simulink model "pwm_sinwave"  (R2015a)
settings: Solver=ode45  StartTime=0.0  StopTime=1  MaxStep=1e-6  RelTol=1e-3
libraries: powerlib x9, simulink x1
settings Model: Creator=KP SINGH  LastModifiedBy=KP SINGH

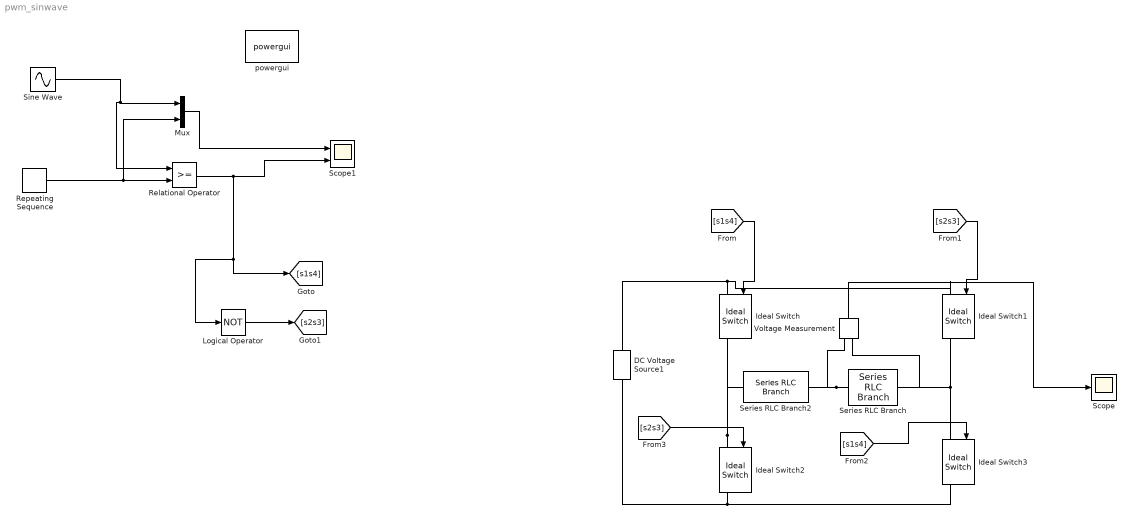
== system pwm_sinwave ==
  DC Voltage Source1 : powerlib/Electrical Sources/DC Voltage Source  Amplitude=100  Measurements=None
  Ideal Switch{,1..3} (4 alike) : powerlib/Power Electronics/Ideal Switch  Ron=0.001  Lon=0  IC=0  Rs=1e5  Cs=inf  Measurements=on
  Logical Operator : Logic  Operator=NOT  IconShape=distinctive  AllPortsSameDT=off  OutDataTypeStr=boolean
  Mux : Mux  Inputs=2
  Relational Operator : RelationalOperator  OutDataTypeStr=boolean
  Repeating Sequence : simulink/Sources/Repeating Sequence  rep_seq_t=[0 1 2 3 4]/10000  rep_seq_y=[0 1 0 -1 0]
  Scope : Scope
      settings: YMin=-100  YMax=100
  Scope1 : Scope  NumInputPorts=2
      settings: YMin=-5~-5  YMax=5~5  MaxDataPoints=5
  Series RLC Branch : powerlib/Elements/Series RLC Branch  LConnTagsString=__new0  RConnTagsString=__new0  BranchType=R  Resistance=100  Inductance=1e-3  SetiL0=off  InitialCurrent=0  Capacitance=1e-6  Setx0=off  InitialVoltage=0  Measurements=None
  Series RLC Branch2 : powerlib/Elements/Series RLC Branch  LConnTagsString=__new0  RConnTagsString=__new0  BranchType=L  Resistance=1  Inductance=50e-3  SetiL0=off  InitialCurrent=0  Capacitance=1e-6  Setx0=off  InitialVoltage=0  Measurements=None
  Sine Wave : Sin  Frequency=2*pi*50  SampleTime=0
  Voltage Measurement : powerlib/Measurements/Voltage Measurement  PhasorSimulation=off  OutputType=Complex  PSBequivalent=0
  powergui : powerlib/powergui  Priority=1  SimulationMode=Continuous  SolverType=Tustin/Backward Euler (TBE)  SampleTime=50e-6  frequency=60  SPID=off  DisableSnubberDevices=off  DisableRonSwitches=off  DisableVfSwitches=off  SwTol=0  DisplayEquations=off  Interpol=off  methode=off  Ts=100  FunctionMessages=off  echomessages=off  HookPort=off  EnableUseOfTLC=off  x0status=blocks  frequencyindice=0  Pbase=100e6  ErrMax=1e-4  Iterations=50  UnitsV=kV  UnitsW=MW  buscounter=0  RestoreLinks=warning  ResistiveCurrentMeasurement=off  Frange=[0:2:500]  Ylog=off  Xlog=on  ShowGrid=off  save=off  variable=ZData  structure=0  ZoomFFT=off  StartTime=0.0  cycles=1  DisplayStyle=1  fundamental=60  FreqAxis=off  MaxFrequency=1000  frequencyindicesteady=1  RmsSteady=1  display=off
  wires:
  Sine Wave/1 -> Relational Operator/1, Mux/1
  Repeating Sequence/1 -> Mux/2, Relational Operator/2
  Mux/1 -> Scope1/1
  Relational Operator/1 -> [s1s4], Logical Operator/1, Scope1/2
  Logical Operator/1 -> [s2s3]
  Voltage Measurement/1 -> Scope/1
  [s2s3] -> Ideal Switch1/1
  [s1s4] -> Ideal Switch/1
  [s2s3] -> Ideal Switch2/1
  [s1s4] -> Ideal Switch3/1
  connections:
  Ideal Switch2/LConn1 -- Series RLC Branch2/LConn1 -- Ideal Switch/RConn1
  Ideal Switch1/RConn1 -- Ideal Switch3/LConn1 -- Voltage Measurement/LConn2 -- Series RLC Branch/RConn1
  Series RLC Branch/LConn1 -- Series RLC Branch2/RConn1 -- Voltage Measurement/LConn1
  Ideal Switch2/RConn1 -- Ideal Switch3/RConn1 -- DC Voltage Source1/LConn1
  Ideal Switch/LConn1 -- DC Voltage Source1/RConn1 -- Ideal Switch1/LConn1
